simulink model "HeatExchanger_digital_sanity"  (R2013a)
settings: Solver=ode4  StartTime=0.0  StopTime=250  FixedStep=delta_t  RelTol=1e-3
values from neighbouring files (symbols this model uses):
  Ts = delta_t    (= 0.1)    [HeatExchanger_ps.m]    (also in hxpumpcode.m = params.Ts; hxpumpcodesanity.m; noErrornoDelay.mat)
libraries: simulink x4
settings Model: Creator=Rhine  LastModifiedBy=LabUser
settings DataIOCC: LimitDataPoints=off  SignalLoggingSaveFormat=ModelDataLogs
settings OptimizationCC: ExpressionDepthLimit=2147483647
settings DebuggingCC: FcnCallInpInsideContextMsg=UseLocalSettings
settings GRTTargetCC: CodeReplacementLibrary=None  CombineOutputUpdateFcns=off  CPPClassGenCompliant=on  GRTInterface=on

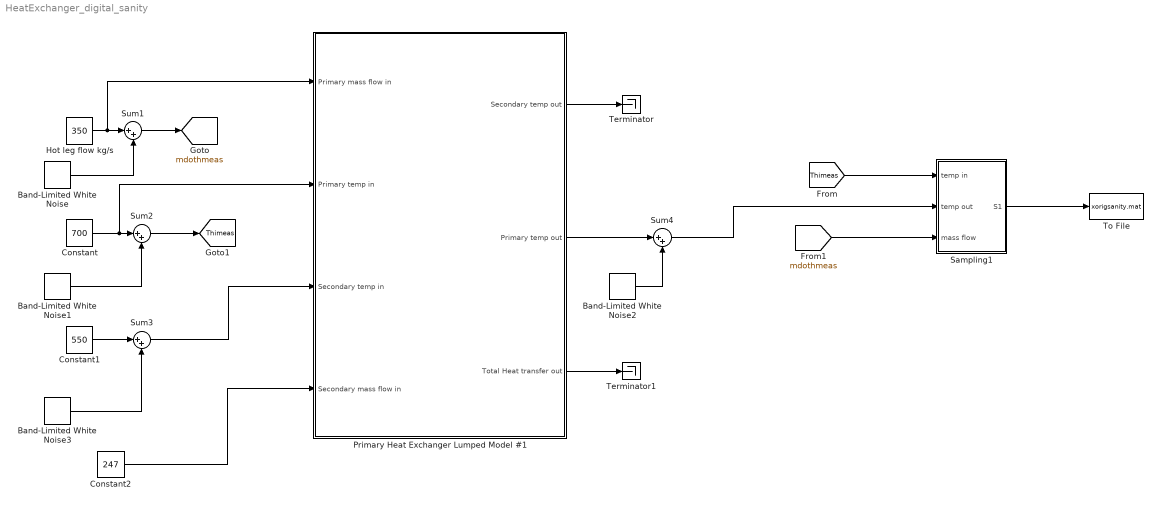
== system HeatExchanger_digital_sanity ==
  Band-Limited White Noise : simulink/Sources/Band-Limited White Noise  Cov=0  Ts=Ts  seed=[34567]
  Band-Limited White Noise1 : simulink/Sources/Band-Limited White Noise  Cov=0  Ts=Ts  seed=[11111]
  Band-Limited White Noise2 : simulink/Sources/Band-Limited White Noise  Cov=0  Ts=Ts  seed=[45678]
  Band-Limited White Noise3 : simulink/Sources/Band-Limited White Noise  Cov=0  Ts=Ts  seed=[23341]
  Constant : Constant  Value=700
  Constant1 : Constant  Value=550
  Constant2 : Constant  Value=247
  Hot leg flow kg/s : Constant  Value=350
  Primary Heat Exchanger Lumped Model #1 : Subsystem
  Sampling1 : Subsystem
  Sum{1..4} (4 alike) : Sum  Inputs=|++
  Terminator : Terminator
  Terminator1 : Terminator
  To File : ToFile  Filename=xorigsanity.mat  MatrixName=xorigsanity
  tag scope: Thimeas=global, mdothmeas=global
  wires:
  Hot leg flow kg/s/1 -> Primary Heat Exchanger Lumped Model #1/1(Primary mass flow in), Sum1/1
  Constant/1 -> Primary Heat Exchanger Lumped Model #1/2(Primary temp in), Sum2/1
  Constant1/1 -> Sum3/1
  Sum3/1 -> Primary Heat Exchanger Lumped Model #1/3(Secondary temp in)
  Primary Heat Exchanger Lumped Model #1/1(Secondary temp out) -> Terminator/1
  Primary Heat Exchanger Lumped Model #1/3("Total Heat transfer out ") -> Terminator1/1
  Sum1/1 -> [mdothmeas]
  Sum2/1 -> [Thimeas]
  [Thimeas] -> Sampling1/1(temp in)
  [mdothmeas] -> Sampling1/3(mass flow)
  Primary Heat Exchanger Lumped Model #1/2(Primary temp out) -> Sum4/1
  Band-Limited White Noise/1 -> Sum1/2
  Band-Limited White Noise1/1 -> Sum2/2
  Band-Limited White Noise2/1 -> Sum4/2
  Sum4/1 -> Sampling1/2(temp out)
  Band-Limited White Noise3/1 -> Sum3/2
  Constant2/1 -> Primary Heat Exchanger Lumped Model #1/4(Secondary mass flow in)
  Sampling1/1(S1) -> To File/1

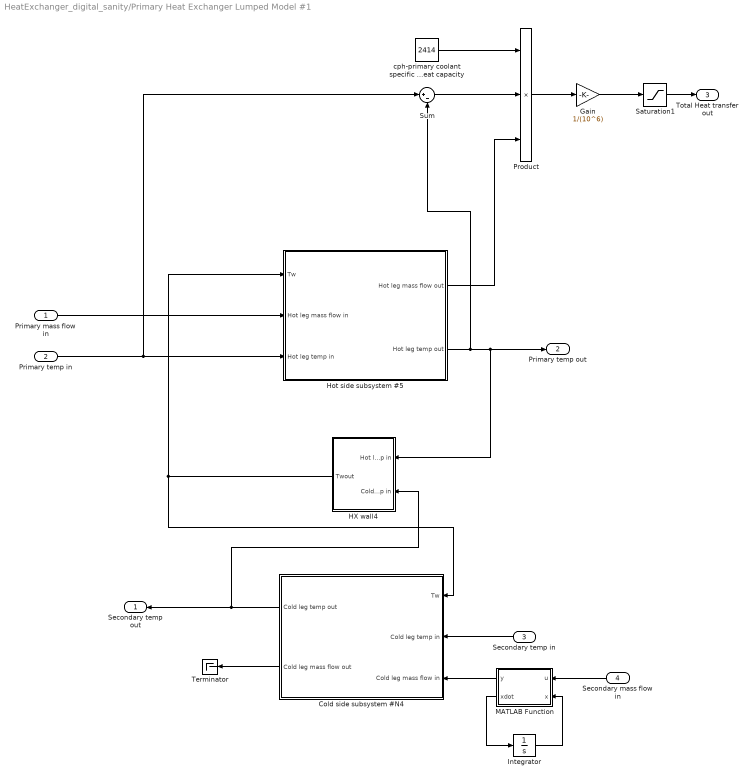
== system HeatExchanger_digital_sanity/Primary Heat Exchanger Lumped Model #1 ==
  Primary mass flow in : Inport
  Primary temp in : Inport  Port=2
  Secondary temp in : Inport  Port=3
  Secondary mass flow in : Inport  Port=4
  Cold side subsystem #N4 : Subsystem
  Gain : Gain  Gain=1/(10^6)
  HX wall4 : Subsystem
  Hot side subsystem #5 : Subsystem
  Integrator : Integrator  InitialCondition=250
  MATLAB Function : MATLAB Function  TreatAsAtomicUnit=on
  Product : Product  Inputs=3
  Saturation1 : Saturate  UpperLimit=inf  LowerLimit=0
  Sum : Sum  Inputs=|+-
  Terminator : Terminator
  cph-primary coolant specific heat capacity : Constant  Value=2414
  Secondary temp out : Outport
  Primary temp out : Outport  Port=2
  "Total Heat transfer out " : Outport  Port=3
  wires:
  Cold side subsystem #N4/1(Cold leg temp out) -> Secondary temp out/1, HX wall4/2(Cold leg temp in)
  Cold side subsystem #N4/2(Cold leg mass flow out) -> Terminator/1
  Primary mass flow in/1 -> Hot side subsystem #5/2(Hot leg mass flow in)
  Primary temp in/1 -> Hot side subsystem #5/3(Hot leg temp in), Sum/1
  Secondary mass flow in/1 -> MATLAB Function/1(u)
  Secondary temp in/1 -> Cold side subsystem #N4/2(Cold leg temp in)
  HX wall4/1(Twout) -> Cold side subsystem #N4/1(Tw), Hot side subsystem #5/1(Tw)
  Hot side subsystem #5/1(Hot leg mass flow out) -> Product/3
  Hot side subsystem #5/2(Hot leg temp out) -> HX wall4/1(Hot leg temp in), Primary temp out/1, Sum/2
  cph-primary coolant specific heat capacity/1 -> Product/1
  Sum/1 -> Product/2
  Product/1 -> Gain/1
  Gain/1 -> Saturation1/1
  MATLAB Function/1(y) -> Cold side subsystem #N4/3(Cold leg mass flow in)
  Saturation1/1 -> "Total Heat transfer out "/1
  MATLAB Function/2(xdot) -> Integrator/1
  Integrator/1 -> MATLAB Function/2(x)

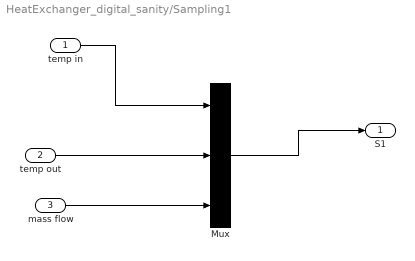
== system HeatExchanger_digital_sanity/Sampling1 ==
  temp in : Inport
  temp out : Inport  Port=2
  mass flow : Inport  Port=3
  Mux : Mux  Inputs=3
  S1 : Outport
  wires:
  temp in/1 -> Mux/1
  temp out/1 -> Mux/2
  mass flow/1 -> Mux/3
  Mux/1 -> S1/1

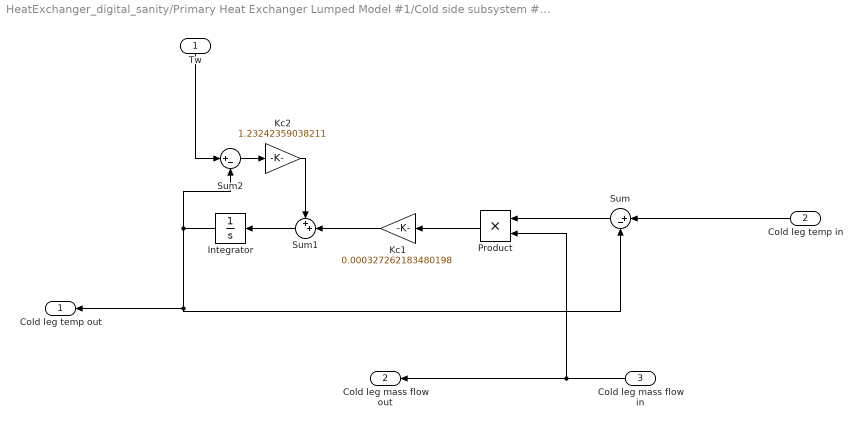
== system HeatExchanger_digital_sanity/Primary Heat Exchanger Lumped Model #1/Cold side subsystem #N4 ==
  Tw : Inport
  Cold leg temp in : Inport  Port=2
  Cold leg mass flow in : Inport  Port=3
  Integrator : Integrator  InitialCondition=638.4
  Kc1 : Gain  Gain=0.000327262183480198
  Kc2 : Gain  Gain=1.23242359038211
  Product : Product
  Sum : Sum  Inputs=|+-
  Sum1 : Sum  Inputs=++|
  Sum2 : Sum  Inputs=|+-
  Cold leg temp out : Outport
  Cold leg mass flow out : Outport  Port=2
  wires:
  Cold leg temp in/1 -> Sum/1
  Integrator/1 -> Sum/2, Cold leg temp out/1, Sum2/2
  Sum2/1 -> Kc2/1
  Sum/1 -> Product/1
  Kc2/1 -> Sum1/1
  Sum1/1 -> Integrator/1
  Cold leg mass flow in/1 -> Cold leg mass flow out/1, Product/2
  Product/1 -> Kc1/1
  Kc1/1 -> Sum1/2
  Tw/1 -> Sum2/1

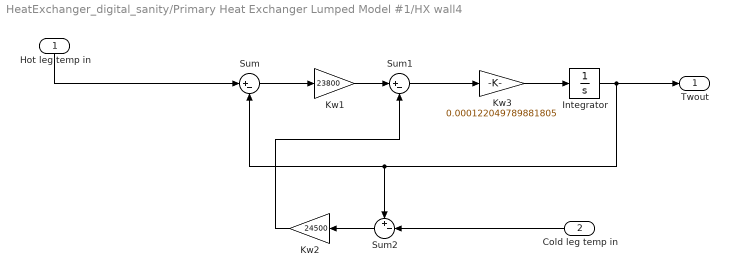
== system HeatExchanger_digital_sanity/Primary Heat Exchanger Lumped Model #1/HX wall4 ==
  Hot leg temp in : Inport
  Cold leg temp in : Inport  Port=2
  Integrator : Integrator  InitialCondition=644.3
  Kw1 : Gain  Gain=23800
  Kw2 : Gain  Gain=24500
  Kw3 : Gain  Gain=0.000122049789881805
  Sum : Sum  Inputs=|+-
  Sum1 : Sum  Inputs=|+-
  Sum2 : Sum  Inputs=+-|
  Twout : Outport
  wires:
  Sum2/1 -> Kw2/1
  Hot leg temp in/1 -> Sum/1
  Sum1/1 -> Kw3/1
  Cold leg temp in/1 -> Sum2/2
  Sum/1 -> Kw1/1
  Kw1/1 -> Sum1/1
  Kw3/1 -> Integrator/1
  Integrator/1 -> Twout/1, Sum2/1, Sum/2
  Kw2/1 -> Sum1/2

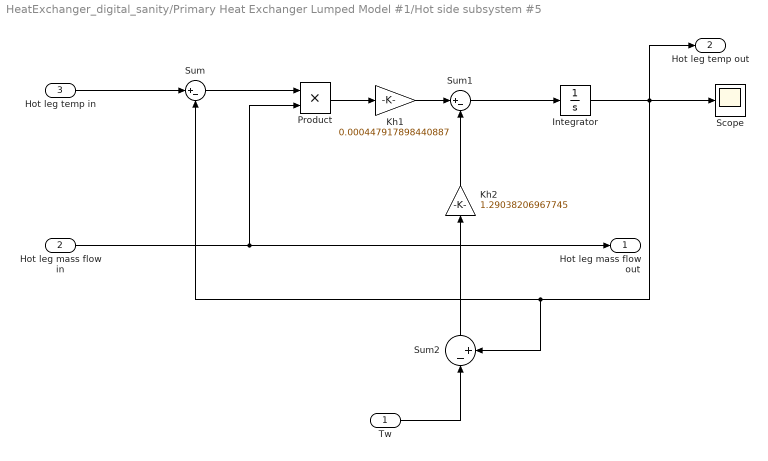
== system HeatExchanger_digital_sanity/Primary Heat Exchanger Lumped Model #1/Hot side subsystem #5 ==
  Tw : Inport
  Hot leg mass flow in : Inport  Port=2
  Hot leg temp in : Inport  Port=3
  Integrator : Integrator  InitialCondition=650.29
  Kh1 : Gain  Gain=0.000447917898440887
  Kh2 : Gain  Gain=1.29038206967745
  Product : Product
  Scope : Scope
  Sum : Sum  Inputs=|+-
  Sum1 : Sum  Inputs=|+-
  Sum2 : Sum  Inputs=|-+
  Hot leg mass flow out : Outport
  Hot leg temp out : Outport  Port=2
  wires:
  Product/1 -> Kh1/1
  Kh1/1 -> Sum1/1
  Sum1/1 -> Integrator/1
  Sum2/1 -> Kh2/1
  Kh2/1 -> Sum1/2
  Tw/1 -> Sum2/1
  Hot leg temp in/1 -> Sum/1
  Hot leg mass flow in/1 -> Hot leg mass flow out/1, Product/2
  Sum/1 -> Product/1
  Integrator/1 -> Hot leg temp out/1, Scope/1, Sum2/2, Sum/2

== matlab function HeatExchanger_digital_sanity/Primary Heat Exchanger Lumped Model #1/MATLAB Function ==
  data: u input; y output; x input; xdot output
function [y,xdot] = pump(u,x)
%#codegen

if u<0
    u=0;
else
end

xdot = -0.1*x + 0.1*u;

y = x;
